simulink model "mod_ps"  (R2021b)
settings: Solver=FixedStepAuto  StartTime=0.0  StopTime=2300  FixedStep=1e-3  RelTol=1e-3
settings Model: Creator=lucas  LastModifiedBy=lucas

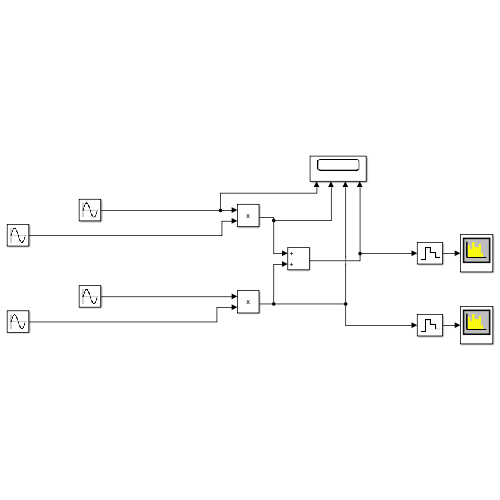
[thumbnail: Simulink's stored preview of the top-level diagram]
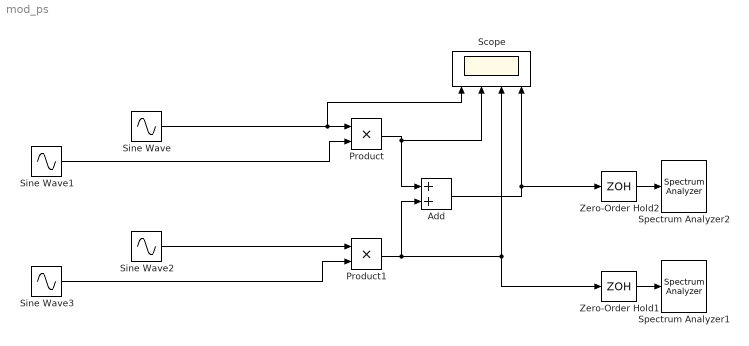
== system mod_ps ==
  Add : Sum
  Product : Product
  Product1 : Product
  Scope : Scope  NumInputPorts=4
  Sine Wave : Sin  Amplitude=2  Frequency=2*pi*2  Phase=-(pi/2)  SampleTime=0
  Sine Wave1 : Sin  Amplitude=2  Frequency=2*pi*20  SampleTime=0
  Sine Wave2 : Sin  Amplitude=2  Frequency=2*pi*2  SampleTime=0
  Sine Wave3 : Sin  Amplitude=2  Frequency=2*pi*20  Phase=-(pi/2)  SampleTime=0
  Spectrum Analyzer1 : SpectrumAnalyzer
  Spectrum Analyzer2 : SpectrumAnalyzer
  Zero-Order Hold1 : ZeroOrderHold  SampleTime=-1
  Zero-Order Hold2 : ZeroOrderHold  SampleTime=-1
  wires:
  Product/1 -> Scope/2, Add/1
  Product1/1 -> Zero-Order Hold1/1, Scope/3, Add/2
  Sine Wave1/1 -> Product/2
  Sine Wave3/1 -> Product1/2
  Sine Wave2/1 -> Product1/1
  Sine Wave/1 -> Scope/1, Product/1
  Add/1 -> Zero-Order Hold2/1, Scope/4
  Zero-Order Hold2/1 -> Spectrum Analyzer2/1
  Zero-Order Hold1/1 -> Spectrum Analyzer1/1
